simulink model "BirdEyeView_NN"  (R2022a)
settings: Solver=FixedStepDiscrete  StartTime=0.0  StopTime=Ts_480p*4  RelTol=1e-3
InitFcn:
  | Ts = 1e-3;
  | Ts_240p = 402*324*Ts;
  | Ts_480p = 525*800*Ts;
  | global lut;
  | %temp = load('lut_rc_c.mat');
  | %lut = temp.lut_rc_c;
undefined symbols (not defined in the file or in its folder): gray, Rec, SDTV
libraries: hdlsllib x10, visionhdlio x2, visionhdlconversions x1, dspvision x1
settings Model: DataTypeOverride=Off  ModifiedByFormat=4mbilal@gmail.com  Creator=The MathWorks, Inc.  LastModifiedBy=4mbilal@gmail.com
settings SolverCC: AlgebraicLoopSolver=TrustRegion
settings DataIOCC: LimitDataPoints=on  SaveFormat=Array  SaveOutput=off  SaveTime=off  ReturnWorkspaceOutputs=off
settings OptimizationCC: BlockReduction=off  ConditionallyExecuteInputs=off  DefaultParameterBehavior=Inlined  LifeSpan=inf
settings DebuggingCC: AlgebraicLoopMsg=error  SolverPrmCheckMsg=warning  SingleTaskRateTransMsg=error  ParameterPrecisionLossMsg=none  UnconnectedInputMsg=warning  UnconnectedOutputMsg=warning  UnconnectedLineMsg=warning  AllowSymbolicDim=off  SFUnexpectedBacktrackingDiag=warning  SFNoUnconditionalDefaultTransitionDiag=warning  SFExecutionAtInitializationDiag=none  SFMachineParentedDataDiag=warning  IntegerSaturationMsg=none  ArithmeticOperatorsInVariantConditions=warning
settings HardwareCC: ProdBitPerPointer=32  ProdBitPerSizeT=32  ProdBitPerPtrDiffT=32  ProdLargestAtomicFloat=None  ProdIntDivRoundTo=Undefined  ProdEndianess=Unspecified  ProdWordSize=32  ProdHWDeviceType=ASIC/FPGA->ASIC/FPGA  ProdEqTarget=off
settings ModelReferenceCC: PropagateSignalLabelsOutOfModel=off
settings SFSimCC: SimUseLocalCustomCode=off  CustomCodeUndefinedFunction=UseInterfaceOnly
settings RTWCC: RTWUseLocalCustomCode=off
settings CodeAppCC: StateflowObjectComments=on
settings GRTTargetCC: TargetLangStandard=C89/C90 (ANSI)
settings ConfigComp: CovMetricSettings=dw  CovSaveCumulativeToWorkspaceVar=on  CovSaveSingleToWorkspaceVar=on  CovExternalEMLEnable=off  CovSFcnEnable=off

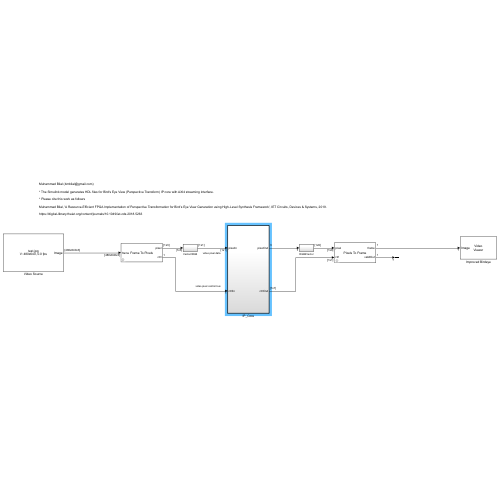
[thumbnail: Simulink's stored preview of the top-level diagram]
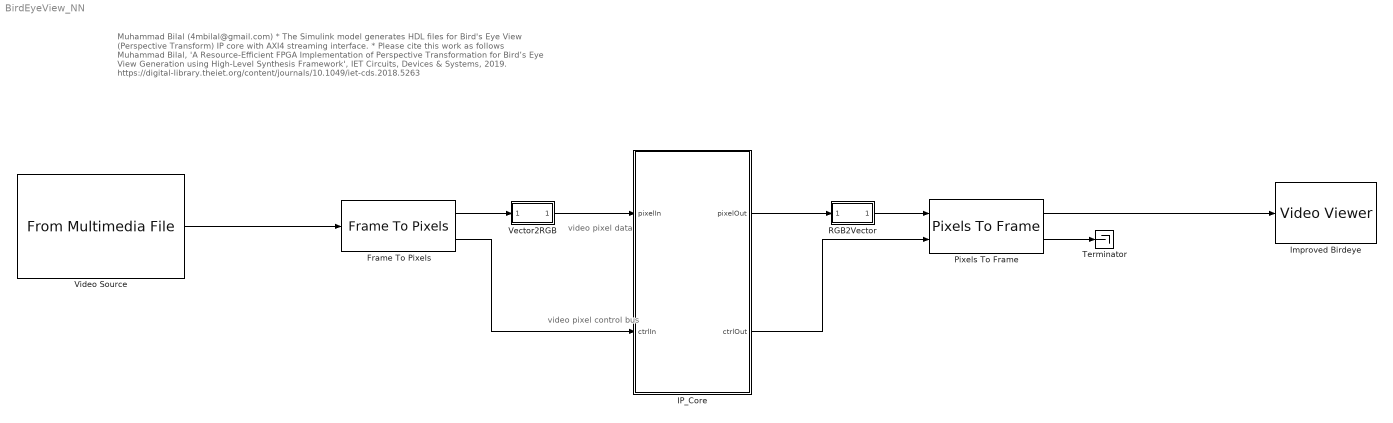
== system BirdEyeView_NN ==
  note: Muhammad Bilal (4mbilal@gmail.com)
      |
      | * The Simulink model generates HDL files for Bird's Eye View (Perspective Transform) IP core with AXI4 streaming interface.
      |
      | * Please cite this work as follows
      |
      | Muhammad Bilal, 'A Resource-Efficient FPGA Implementation of Perspective Transformation for Bird’s Eye View Generation using High-Level Synthesis Framework', IET Circuits, Devices & Systems, 2019.
      |
      | https://digital-library.theiet.org/content/journals/10.1049/iet-cds.2018.5263
  note: video pixel data
  note: video pixel control bus
  Frame To Pixels : visionhdlio/Frame To Pixels  NumComponents=3  NumPixels=1  VideoFormat=480p  ActivePixelsPerLine=640  ActiveVideoLines=480  TotalPixelsPerLine=800  TotalVideoLines=525  StartingActiveLine=36  FrontPorch=16  SampleTime=0  VideoFormatCache=480p  ActivePixelsPerLineCache=32  ActiveVideoLinesCache=18  TotalPixelsPerLineCache=42  TotalVideoLinesCache=28  StartingActiveLineCache=6  FrontPorchCache=5
      settings: SourceProductBaseCode=VT
  IP_Core : Subsystem  TreatAsAtomicUnit=on
  Improved Birdeye : VideoViewer  colormapValue=gray(256)  FigPos=[1 822 1536 724]
  Pixels To Frame : visionhdlio/Pixels To Frame  NumComponents=3  NumPixels=1  VideoFormat=480p  ActivePixelsPerLine=640  ActiveVideoLines=480  TotalPixelsPerLine=800  TotalVideoLines=525  VideoFormatCache=480p  ActivePixelsPerLineCache=32  ActiveVideoLinesCache=18  TotalPixelsPerLineCache=42  TotalVideoLinesCache=28
      settings: SourceProductBaseCode=VT
  RGB2Vector : Subsystem
  Terminator : Terminator
  Vector2RGB : Subsystem
  Video Source : dspvision/From Multimedia File  inputFilename=D:\Zedboard\custom_ip_cores\Mathworks\BirdsEyeView\test.jpg  readRange=[1 Inf]  loop=on  numPlays=inf  outputStreams=Video only  videoDataType=uint8  audioDataType=int16  inheritSampleTime=off  userDefinedSampleTime=Ts_480p  noAudioOutput=off  isIntensityVideo=off  fourcc=RGB  colorVideoFormat=One multidimensional signal  outputEOF=off  dataOrg=Column-major  audioFrameSize=1024  computeAudioFrameSize=off  outSamplingMode=Sample based
  wires:
  Pixels To Frame/2 -> Terminator/1
  Vector2RGB/1(RGB) -> IP_Core/1(pixelIn)
  IP_Core/1(pixelOut) -> RGB2Vector/1(RGB)
  Frame To Pixels/1 -> Vector2RGB/1(RGBVector)
  IP_Core/2(ctrlOut) -> Pixels To Frame/2
  Frame To Pixels/2 -> IP_Core/2(ctrlIn)
  RGB2Vector/1(RGBVector) -> Pixels To Frame/1
  Pixels To Frame/1 -> Improved Birdeye/1
  Video Source/1 -> Frame To Pixels/1

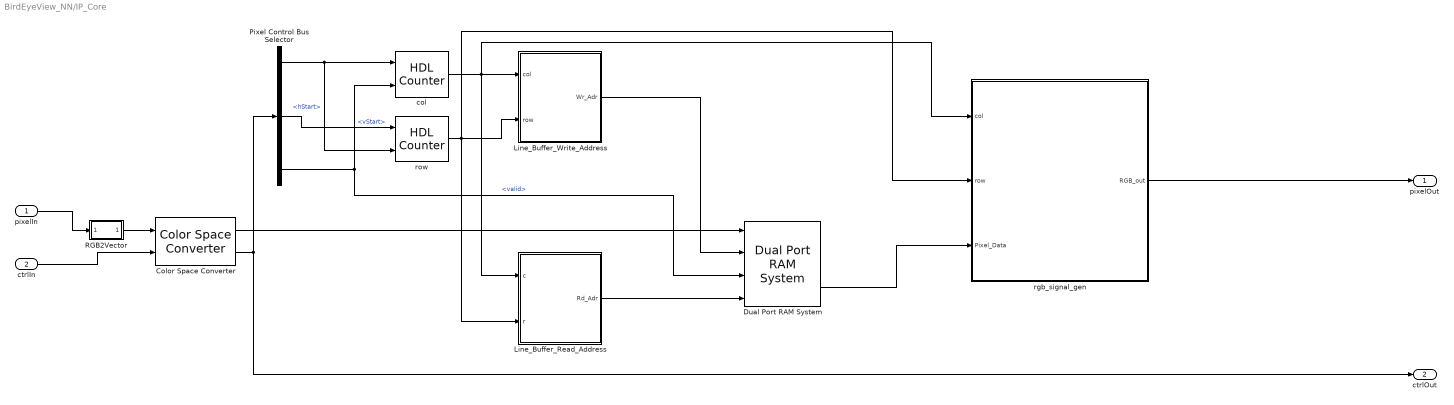
== system BirdEyeView_NN/IP_Core ==
  pixelIn : Inport
  ctrlIn : Inport  Port=2
  Color Space Converter : visionhdlconversions/Color Space Converter  Conversion=RGB to intensity  ConversionStandard=Rec. 601 (SDTV)  ScanningStandard=1250/50/2:1  SimulateUsing=Code generation
      settings: SourceProductBaseCode=VT
  Dual Port RAM System : hdlsllib/HDL RAMs/Dual Port RAM System  RAMType=Dual port  WriteOutputValue=New data  RAMInitialValue=0  SimulateUsing=Code generation
      settings: SourceProductBaseCode=SL
  Line_Buffer_Read_Address : MATLAB Function  TreatAsAtomicUnit=on
  Line_Buffer_Write_Address : MATLAB Function  TreatAsAtomicUnit=on
  Pixel Control Bus Selector : BusSelector  OutputSignals=hStart,hEnd,vStart,vEnd,valid
  RGB2Vector : Subsystem
  col : hdlsllib/Sources/HDL Counter  CountType=Count limited  CountInit=0  CountStep=1  CountMax=638  CountFromType=Initial value  CountFrom=0  CountResetPort=on  CountLoadPort=off  CountEnbPort=on  CountDirPort=off  CountHitOutputPort=off  CountDataType=Unsigned  CountWordLen=10  CountFracLen=0  CountSampTime=1
  rgb_signal_gen : MATLAB Function  TreatAsAtomicUnit=on
  row : hdlsllib/Sources/HDL Counter  CountType=Count limited  CountInit=0  CountStep=1  CountMax=638  CountFromType=Initial value  CountFrom=0  CountResetPort=on  CountLoadPort=off  CountEnbPort=on  CountDirPort=off  CountHitOutputPort=off  CountDataType=Unsigned  CountWordLen=10  CountFracLen=0  CountSampTime=1
  pixelOut : Outport  VectorParamsAs1DForOutWhenUnconnected=off
  ctrlOut : Outport  Port=2  VectorParamsAs1DForOutWhenUnconnected=off
  wires:
  ctrlIn/1 -> Color Space Converter/2
  pixelIn/1 -> RGB2Vector/1(RGB)
  RGB2Vector/1(RGBVector) -> Color Space Converter/1
  rgb_signal_gen/1(RGB_out) -> pixelOut/1
  Color Space Converter/2 -> ctrlOut/1, Pixel Control Bus Selector/1
  Pixel Control Bus Selector/1 -> row/2, col/1  "<hStart>"
  col/1 -> rgb_signal_gen/1(col), Line_Buffer_Read_Address/1(c), Line_Buffer_Write_Address/1(col)
  Pixel Control Bus Selector/5 -> col/2, Dual Port RAM System/3  "<valid>"
  Line_Buffer_Read_Address/1(Rd_Adr) -> Dual Port RAM System/4
  Pixel Control Bus Selector/3 -> row/1  "<vStart>"
  row/1 -> Line_Buffer_Read_Address/2(r), rgb_signal_gen/2(row), Line_Buffer_Write_Address/2(row)
  Color Space Converter/1 -> Dual Port RAM System/1
  Line_Buffer_Write_Address/1(Wr_Adr) -> Dual Port RAM System/2
  Dual Port RAM System/2 -> rgb_signal_gen/3(Pixel_Data)

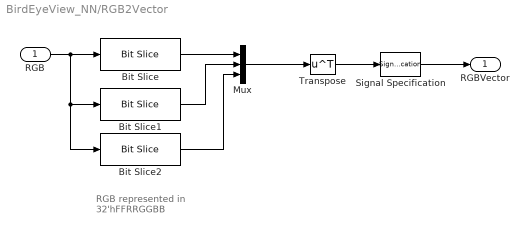
== system BirdEyeView_NN/RGB2Vector ==
  note: RGB represented in
      | 32'hFFRRGGBB
  RGB : Inport
  Bit Slice : hdlsllib/Logic and Bit Operations/Bit Slice  lidx=23  ridx=16
      settings: SourceProductBaseCode=SL
  Bit Slice1 : hdlsllib/Logic and Bit Operations/Bit Slice  lidx=15  ridx=8
      settings: SourceProductBaseCode=SL
  Bit Slice2 : hdlsllib/Logic and Bit Operations/Bit Slice  lidx=7  ridx=0
      settings: SourceProductBaseCode=SL
  Mux : Mux  Inputs=3
  Signal Specification : SignalSpecification
  Transpose : Math  Operator=transpose  SignedPower=on
  RGBVector : Outport  VectorParamsAs1DForOutWhenUnconnected=off
  wires:
  Mux/1 -> Transpose/1
  Bit Slice/1 -> Mux/1
  Bit Slice2/1 -> Mux/3
  Bit Slice1/1 -> Mux/2
  RGB/1 -> Bit Slice2/1, Bit Slice1/1, Bit Slice/1
  Transpose/1 -> Signal Specification/1
  Signal Specification/1 -> RGBVector/1

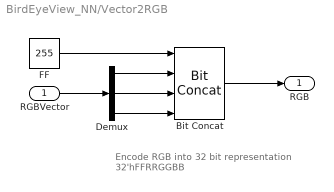
== system BirdEyeView_NN/Vector2RGB ==
  note: Encode RGB into 32 bit representation
      | 32'hFFRRGGBB
  RGBVector : Inport
  Bit Concat : hdlsllib/Logic and Bit Operations/Bit Concat  numInputs=4
  Demux : Demux  Outputs=3
  FF : Constant  Value=255  OutDataTypeStr=uint8  SampleTime=Ts
  RGB : Outport  VectorParamsAs1DForOutWhenUnconnected=off
  wires:
  Bit Concat/1 -> RGB/1
  RGBVector/1 -> Demux/1
  FF/1 -> Bit Concat/1
  Demux/1 -> Bit Concat/2
  Demux/2 -> Bit Concat/3
  Demux/3 -> Bit Concat/4

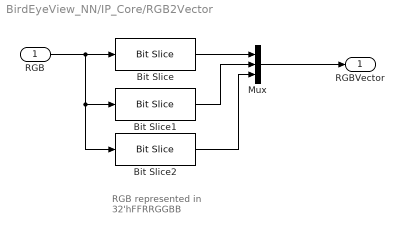
== system BirdEyeView_NN/IP_Core/RGB2Vector ==
  note: RGB represented in
      | 32'hFFRRGGBB
  RGB : Inport
  Bit Slice : hdlsllib/Logic and Bit Operations/Bit Slice  lidx=23  ridx=16
      settings: SourceProductBaseCode=SL
  Bit Slice1 : hdlsllib/Logic and Bit Operations/Bit Slice  lidx=15  ridx=8
      settings: SourceProductBaseCode=SL
  Bit Slice2 : hdlsllib/Logic and Bit Operations/Bit Slice  lidx=7  ridx=0
      settings: SourceProductBaseCode=SL
  Mux : Mux  Inputs=3
  RGBVector : Outport  VectorParamsAs1DForOutWhenUnconnected=off
  wires:
  Bit Slice/1 -> Mux/1
  Bit Slice2/1 -> Mux/3
  Bit Slice1/1 -> Mux/2
  RGB/1 -> Bit Slice2/1, Bit Slice1/1, Bit Slice/1
  Mux/1 -> RGBVector/1

== matlab function BirdEyeView_NN/IP_Core/Line_Buffer_Read_Address ==
  data: c input; Rd_Adr output; r input
function Rd_Adr  = rd_adr_gen(c,r)
% r_in = double(r);
% c_in = double(c);

% col_adr = (216.3 - 0.06823*r_in + 0.3218*c_in - 0.000236*r_in^2 + 0.0002136*r_in*c_in + 0.0000007421*r_in^2*c_in);
% row_adr = (196.8 + 0.01674*r_in + 5.779e-05*r_in^2);


% Fixed-point 24-bit implementation
r_in = fi(r);
c_in = fi(c);

c1 = fi(216.3);
c2 = fi(-0.06823);
c3 = fi(0.3218);
c4 = fi(-0.000236);
c5 = fi(0.0002136);
c6 = fi(0.0000007421);
col_adr = (c1 + c2*r_in + c3*c_in + c4*r_in^2 + c5*r_in*c_in + c6*r_in^2*c_in);

% r1 = fi(196.8);
r1 = fi(0.8);
r2 = fi(0.01674);
r3 = fi(5.779e-05);
row_adr = (r1 + r2*r_in + r3*r_in^2);

col_adr_fi = fi(col_adr, 0, 10, 0);
row_adr_fi = fi(row_adr, 0, 9, 0);

full_adr = row_adr_fi*640 + col_adr_fi;

Rd_Adr = fi(full_adr, 0, 14, 0);%convert to fixed-point 14-bit signal

== matlab function BirdEyeView_NN/IP_Core/rgb_signal_gen ==
  data: col input; row input; Pixel_Data input; RGB_out output
function RGB_out  = rgb_signal_gen(col,row,Pixel_Data)

in_d = double(Pixel_Data);%Double precision format
% if(row<196)
%     in_d = 0;
% elseif(row>430)
%     in_d = 0;
% end
% if(col<50)
%     in_d = 0;
% elseif(col>590)
%     in_d = 0;
% end

R = fi(in_d, 0, 8, 0);%convert to fixed-point 8-bit signal
G = fi(in_d, 0, 8, 0);
B = fi(in_d, 0, 8, 0);
A = fi(255, 0, 8, 0);

RGB_out = bitconcat(A,R,G,B);%32-bit output signal

== matlab function BirdEyeView_NN/IP_Core/Line_Buffer_Write_Address ==
  data: col input; Wr_Adr output; row input
function Wr_Adr  = Lin_Buf_Wr_Adr(col,row)

row_adr = double(row);
col_adr = double(col);

%The following code ensures that row_adr is always within the range [0 24],
%Row 24 is the dump. 
if((row_adr<196)|(row_adr>219))
    row_adr = 24;
else
    row_adr = row_adr - 196;
end
    
full_adr = row_adr*640 + col_adr;

%Memory Size = 25*640=16000(=2^14)
Wr_Adr = fi(full_adr, 0, 14, 0);%convert to fixed-point 14-bit signal
